simulink model "MCVT_v6_shell"  (R2021b)
settings: Solver=FixedStepAuto  StartTime=0.0  StopTime=1000000  FixedStep=1/fz  RelTol=1e-3
undefined symbols (not defined in the file or in its folder): fz_3
libraries: lib_subframe x71, slrealtimeutilitieslib x30, lib_header x15, slrealtimeiplib x15
(part 1 of 2)
settings Model: Creator=krishnan  LastModifiedBy=jiw19031
settings SolverCC: AlgebraicLoopSolver=TrustRegion
settings DebuggingCC: SFMachineParentedDataDiag=warning

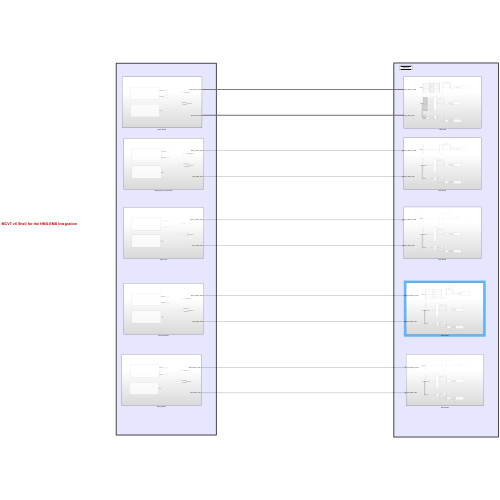
[thumbnail: Simulink's stored preview of the top-level diagram]
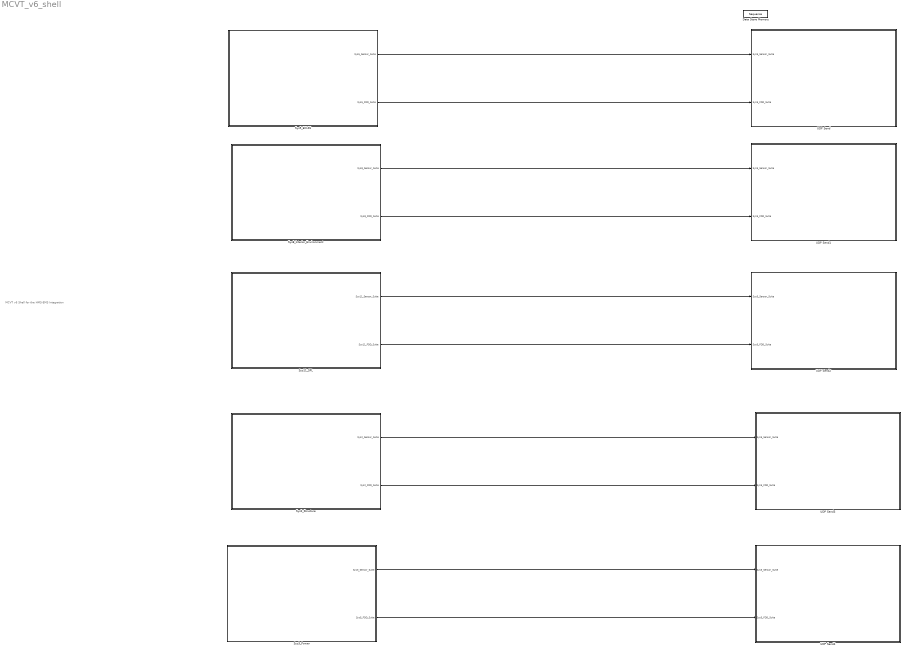
== system MCVT_v6_shell ==
  note: MCVT v6 Shell for the HMS-EMS Integration
  Data Store Memory : DataStoreMemory  DataStoreName=Sequence  ReadBeforeWriteMsg=warning  WriteAfterWriteMsg=warning  WriteAfterReadMsg=warning  ShowAdditionalParam=off  OutDataTypeStr=uint16
  Sys11_SPL : Subsystem
  Sys2_Structure : Subsystem
  Sys3_Power : Subsystem
  Sys5_ECLSS : Subsystem
  Sys8_Interior_Environment : Subsystem
  UDP Send : Subsystem
  UDP Send1 : Subsystem
  UDP Send2 : Subsystem
  UDP Send3 : Subsystem
  UDP Send4 : Subsystem
  wires:
  Sys5_ECLSS/1(Sys5_Sensor_Suite) -> UDP Send/1(Sys5_Sensor_Suite)
  Sys5_ECLSS/2(Sys5_FDD_Suite) -> UDP Send/2(Sys5_FDD_Suite)
  Sys8_Interior_Environment/1(Sys8_Sensor_Suite) -> UDP Send1/1(Sys5_Sensor_Suite)
  Sys8_Interior_Environment/2(Sys8_FDD_Suite) -> UDP Send1/2(Sys5_FDD_Suite)
  Sys11_SPL/1(Sys11_Sensor_Suite) -> UDP Send2/1(Sys5_Sensor_Suite)
  Sys11_SPL/2(Sys11_FDD_Suite) -> UDP Send2/2(Sys5_FDD_Suite)
  Sys2_Structure/1(Sys2_Sensor_Suite) -> UDP Send3/1(Sys5_Sensor_Suite)
  Sys2_Structure/2(Sys2_FDD_Suite) -> UDP Send3/2(Sys5_FDD_Suite)
  Sys3_Power/1(Sys3_Sensor_Suite) -> UDP Send4/1(Sys5_Sensor_Suite)
  Sys3_Power/2(Sys5_FDD_Suite) -> UDP Send4/2(Sys5_FDD_Suite)

== system MCVT_v6_shell/Sys11_SPL ==
  Bus Creator : BusCreator  Inputs=2
  Sys11_FDDs : Subsystem
  Sys11_Sensors : Subsystem
  Sys11_Sensor_Suite : Outport
  Sys11_FDD_Suite : Outport  Port=2
  wires:
  Sys11_Sensors/1(Sys8_Sensor_Measurements) -> [Sys11_Sensor_Suite]
  [Sys11_Sensor_Suite] -> Sys11_Sensor_Suite/1  "Sys11_Sensor_Suite"
  Sys11_Sensors/2(Sys8_Sensor_FDD_Measurements) -> [Sys11_Sensor_FDD]
  Sys11_FDDs/1(Sys11_Component_FDD_Suite) -> [Sys11_Component_FDD]
  [Sys11_Sensor_FDD] -> Bus Creator/1  "Sys11_Sensor_FDD"
  [Sys11_Component_FDD] -> Bus Creator/2  "Sys8_Component_FDD"
  Bus Creator/1 -> Sys11_FDD_Suite/1

== system MCVT_v6_shell/Sys2_Structure ==
  Bus Creator : BusCreator  Inputs=2
  Sys2_FDDs : Subsystem
  Sys2_Sensors : Subsystem
  Sys2_Sensor_Suite : Outport
  Sys2_FDD_Suite : Outport  Port=2
  wires:
  Sys2_Sensors/1(Sys2_Sensor_Measurements) -> [Sys2_Sensor_Suite]
  [Sys2_Sensor_Suite] -> Sys2_Sensor_Suite/1  "Sys2_Sensor_Suite"
  Sys2_Sensors/2(Sys2_Sensor_FDD_Measurements) -> [Sys2_Sensor_FDD]
  Sys2_FDDs/1(Sys2_Component_FDDs) -> [Sys2_Component_FDD]
  [Sys2_Sensor_FDD] -> Bus Creator/1  "Sys2_Sensor_FDD"
  [Sys2_Component_FDD] -> Bus Creator/2  "Sys2_Component_FDD"
  Bus Creator/1 -> Sys2_FDD_Suite/1  "Sys2_FDD_Suite"

== system MCVT_v6_shell/Sys3_Power ==
  Bus Creator : BusCreator  Inputs=2
  Sys3_FDDs : Subsystem
  Sys3_Sensors : Subsystem
  Sys3_Sensor_Suite : Outport
  Sys5_FDD_Suite : Outport  Port=2
  wires:
  Sys3_Sensors/1(Sys3_Sensor_Measurements) -> [Sys3_Sensor_Suite]
  [Sys3_Sensor_Suite] -> Sys3_Sensor_Suite/1  "Sys3_Sensor_Suite"
  Sys3_Sensors/2(Sys3_Sensor_FDD_Measurements) -> [Sys3_Sensor_FDD]
  Sys3_FDDs/1(Sys3_Component_FDDs) -> [Sys3_Component_FDD]
  [Sys3_Sensor_FDD] -> Bus Creator/1  "Sys3_Sensor_FDD"
  [Sys3_Component_FDD] -> Bus Creator/2  "Sys3_Component_FDD"
  Bus Creator/1 -> Sys5_FDD_Suite/1  "Sys3_FDD_Suite"

== system MCVT_v6_shell/Sys5_ECLSS ==
  Bus Creator : BusCreator  Inputs=2
  Sys5_FDDs : Subsystem
  Sys5_Sensors : Subsystem
  Sys5_Sensor_Suite : Outport
  Sys5_FDD_Suite : Outport  Port=2
  wires:
  Sys5_Sensors/1(Sys5_Sensor_Measurements) -> [Sys5_Sensor_Suite]
  [Sys5_Sensor_Suite] -> Sys5_Sensor_Suite/1  "Sys5_Sensor_Suite"
  Sys5_Sensors/2(Sys5_Sensor_FDD_Measurements) -> [Sys5_Sensor_FDD]
  Sys5_FDDs/1(Sys5_Component_FDDs) -> [Sys5_Component_FDD]
  [Sys5_Sensor_FDD] -> Bus Creator/1  "Sys5_Sensor_FDD"
  [Sys5_Component_FDD] -> Bus Creator/2  "Sys5_Component_FDD"
  Bus Creator/1 -> Sys5_FDD_Suite/1  "Sys5_FDD_Suite"

== system MCVT_v6_shell/Sys8_Interior_Environment ==
  Bus Creator : BusCreator  Inputs=2
  Sys8_FDDs : Subsystem
  Sys8_Sensors : Subsystem
  Sys8_Sensor_Suite : Outport
  Sys8_FDD_Suite : Outport  Port=2
  wires:
  Sys8_Sensors/1(Sys8_Sensor_Measurements) -> [Sys8_Sensor_Suite]
  [Sys8_Sensor_Suite] -> Sys8_Sensor_Suite/1  "Sys8_Sensor_Suite"
  Sys8_Sensors/2(Sys8_Sensor_FDD_Measurements) -> [Sys8_Sensor_FDD]
  Sys8_FDDs/1(Sys8_Component_FDD_Suite) -> [Sys8_Component_FDD]
  [Sys8_Sensor_FDD] -> Bus Creator/1  "Sys8_Sensor_FDD"
  [Sys8_Component_FDD] -> Bus Creator/2  "Sys8_Component_FDD"
  Bus Creator/1 -> Sys8_FDD_Suite/1  "Sys8_FDD_Suite"

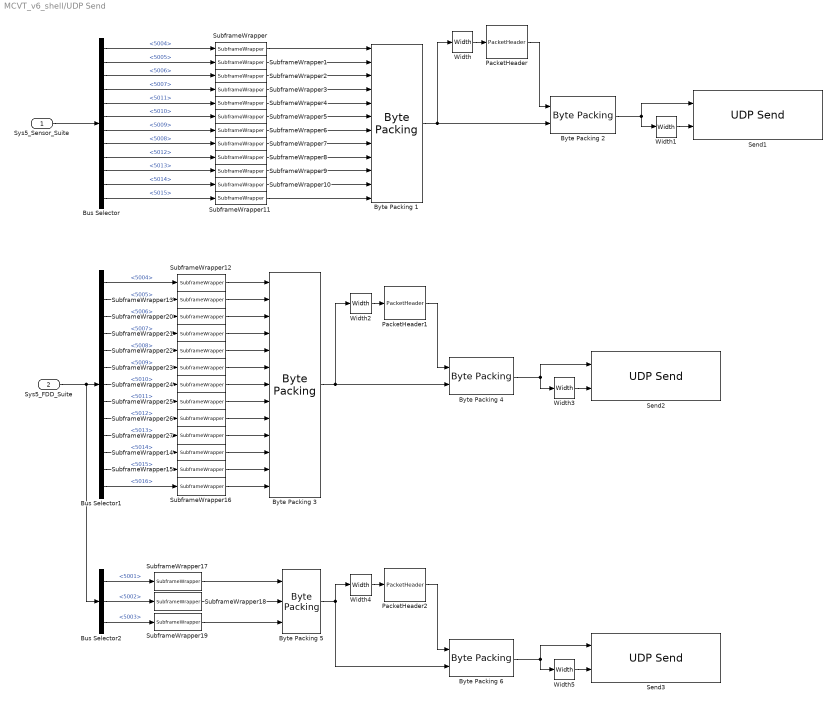
== system MCVT_v6_shell/UDP Send ==
  Sys5_Sensor_Suite : Inport
  Sys5_FDD_Suite : Inport  Port=2
  Bus Selector : BusSelector  OutputSignals=5004,5005,5006,5007,5011,5010,5009,5008,5012,5013,5014,5015
  Bus Selector1 : BusSelector  OutputSignals=Sys5_Sensor_FDD.5004,Sys5_Sensor_FDD.5005,Sys5_Sensor_FDD.5006,Sys5_Sensor_FDD.5007,Sys5_Sensor_FDD.5008,Sys5_Sensor_FDD.5009,Sys5_Sensor_FDD.5010,Sys5_Sensor_FDD.5011,Sys5_Sensor_FDD.5012,Sys5_Sensor_FDD.5013,Sys5_Sensor_FDD.5014,Sys5_Sensor_FDD.5015,Sys5_Sensor_FDD.5016
  Bus Selector2 : BusSelector  OutputSignals=Sys5_Component_FDD.5001,Sys5_Component_FDD.5002,Sys5_Component_FDD.5003
  Byte Packing {1..6} (6 alike) : slrealtimeutilitieslib/Byte Packing
  PacketHeader : lib_header/PacketHeader  src=4  dst=1  pkt_type=1  pkt_priority=1  service=0  flag=0  option1=0  option2=0  subframe_num=12
  PacketHeader1 : lib_header/PacketHeader  src=4  dst=1  pkt_type=1  pkt_priority=1  service=0  flag=0  option1=0  option2=0  subframe_num=13
  PacketHeader2 : lib_header/PacketHeader  src=4  dst=1  pkt_type=1  pkt_priority=1  service=0  flag=0  option1=0  option2=0  subframe_num=3
  Send1 : slrealtimeiplib/UDP Send  useHostTargetConn=on  toAddress=192.168.50.190  toPort=10004  sampleTime=1  localPort=-1
      settings: SourceProductBaseCode=XP
  Send2 : slrealtimeiplib/UDP Send  useHostTargetConn=on  toAddress=192.168.50.190  toPort=10004  sampleTime=1  localPort=-1
      settings: SourceProductBaseCode=XP
  Send3 : slrealtimeiplib/UDP Send  useHostTargetConn=on  toAddress=192.168.50.190  toPort=10004  sampleTime=1  localPort=-1
      settings: SourceProductBaseCode=XP
  SubframeWrapper : lib_subframe/SubframeWrapper  data_id=504
  SubframeWrapper1 : lib_subframe/SubframeWrapper  data_id=505
  SubframeWrapper10 : lib_subframe/SubframeWrapper  data_id=514
  SubframeWrapper11 : lib_subframe/SubframeWrapper  data_id=515
  SubframeWrapper12 : lib_subframe/SubframeWrapper  data_id=5004
  SubframeWrapper13 : lib_subframe/SubframeWrapper  data_id=5005
  SubframeWrapper14 : lib_subframe/SubframeWrapper  data_id=5014
  SubframeWrapper15 : lib_subframe/SubframeWrapper  data_id=5015
  SubframeWrapper16 : lib_subframe/SubframeWrapper  data_id=5016
  SubframeWrapper17 : lib_subframe/SubframeWrapper  data_id=5001
  SubframeWrapper18 : lib_subframe/SubframeWrapper  data_id=5002
  SubframeWrapper19 : lib_subframe/SubframeWrapper  data_id=5003
  SubframeWrapper2 : lib_subframe/SubframeWrapper  data_id=506
  SubframeWrapper20 : lib_subframe/SubframeWrapper  data_id=5006
  SubframeWrapper21 : lib_subframe/SubframeWrapper  data_id=5007
  SubframeWrapper22 : lib_subframe/SubframeWrapper  data_id=5008
  SubframeWrapper23 : lib_subframe/SubframeWrapper  data_id=5009
  SubframeWrapper24 : lib_subframe/SubframeWrapper  data_id=5010
  SubframeWrapper25 : lib_subframe/SubframeWrapper  data_id=5011
  SubframeWrapper26 : lib_subframe/SubframeWrapper  data_id=5012
  SubframeWrapper27 : lib_subframe/SubframeWrapper  data_id=5013
  SubframeWrapper3 : lib_subframe/SubframeWrapper  data_id=507
  SubframeWrapper4 : lib_subframe/SubframeWrapper  data_id=511
  SubframeWrapper5 : lib_subframe/SubframeWrapper  data_id=510
  SubframeWrapper6 : lib_subframe/SubframeWrapper  data_id=509
  SubframeWrapper7 : lib_subframe/SubframeWrapper  data_id=508
  SubframeWrapper8 : lib_subframe/SubframeWrapper  data_id=512
  SubframeWrapper9 : lib_subframe/SubframeWrapper  data_id=513
  Width{,1..5} (6 alike) : Width
  wires:
  Byte Packing 1/1 -> Byte Packing 2/2, Width/1
  Sys5_Sensor_Suite/1 -> Bus Selector/1
  Width/1 -> PacketHeader/1
  PacketHeader/1 -> Byte Packing 2/1
  Byte Packing 2/1 -> Width1/1, Send1/1
  Width1/1 -> Send1/2
  Bus Selector/1 -> SubframeWrapper/1  "<5004>"
  Bus Selector/2 -> SubframeWrapper1/1  "<5005>"
  Bus Selector/3 -> SubframeWrapper2/1  "<5006>"
  Bus Selector/4 -> SubframeWrapper3/1  "<5007>"
  Bus Selector/5 -> SubframeWrapper4/1  "<5011>"
  Bus Selector/6 -> SubframeWrapper5/1  "<5010>"
  Bus Selector/7 -> SubframeWrapper6/1  "<5009>"
  Bus Selector/8 -> SubframeWrapper7/1  "<5008>"
  Bus Selector/9 -> SubframeWrapper8/1  "<5012>"
  Bus Selector/10 -> SubframeWrapper9/1  "<5013>"
  Bus Selector/11 -> SubframeWrapper10/1  "<5014>"
  Bus Selector/12 -> SubframeWrapper11/1  "<5015>"
  SubframeWrapper/1 -> Byte Packing 1/1
  SubframeWrapper1/1 -> Byte Packing 1/2
  SubframeWrapper2/1 -> Byte Packing 1/3
  SubframeWrapper3/1 -> Byte Packing 1/4
  SubframeWrapper4/1 -> Byte Packing 1/5
  SubframeWrapper5/1 -> Byte Packing 1/6
  SubframeWrapper6/1 -> Byte Packing 1/7
  SubframeWrapper7/1 -> Byte Packing 1/8
  SubframeWrapper8/1 -> Byte Packing 1/9
  SubframeWrapper9/1 -> Byte Packing 1/10
  SubframeWrapper10/1 -> Byte Packing 1/11
  SubframeWrapper11/1 -> Byte Packing 1/12
  Bus Selector2/2 -> SubframeWrapper18/1  "<5002>"
  Byte Packing 6/1 -> Width5/1, Send3/1
  SubframeWrapper18/1 -> Byte Packing 5/2
  Bus Selector1/8 -> SubframeWrapper25/1  "<5011>"
  PacketHeader2/1 -> Byte Packing 6/1
  SubframeWrapper17/1 -> Byte Packing 5/1
  Bus Selector1/11 -> SubframeWrapper14/1  "<5014>"
  SubframeWrapper14/1 -> Byte Packing 3/11
  SubframeWrapper27/1 -> Byte Packing 3/10
  Bus Selector1/4 -> SubframeWrapper21/1  "<5007>"
  SubframeWrapper19/1 -> Byte Packing 5/3
  SubframeWrapper15/1 -> Byte Packing 3/12
  SubframeWrapper16/1 -> Byte Packing 3/13
  Bus Selector2/3 -> SubframeWrapper19/1  "<5003>"
  Byte Packing 5/1 -> Byte Packing 6/2, Width4/1
  SubframeWrapper25/1 -> Byte Packing 3/8
  Width4/1 -> PacketHeader2/1
  SubframeWrapper26/1 -> Byte Packing 3/9
  Bus Selector2/1 -> SubframeWrapper17/1  "<5001>"
  Bus Selector1/7 -> SubframeWrapper24/1  "<5010>"
  SubframeWrapper12/1 -> Byte Packing 3/1
  Bus Selector1/10 -> SubframeWrapper27/1  "<5013>"
  Bus Selector1/9 -> SubframeWrapper26/1  "<5012>"
  Bus Selector1/12 -> SubframeWrapper15/1  "<5015>"
  Byte Packing 3/1 -> Byte Packing 4/2, Width2/1
  Bus Selector1/13 -> SubframeWrapper16/1  "<5016>"
  SubframeWrapper24/1 -> Byte Packing 3/7
  SubframeWrapper23/1 -> Byte Packing 3/6
  SubframeWrapper21/1 -> Byte Packing 3/4
  SubframeWrapper20/1 -> Byte Packing 3/3
  Bus Selector1/2 -> SubframeWrapper13/1  "<5005>"
  SubframeWrapper22/1 -> Byte Packing 3/5
  SubframeWrapper13/1 -> Byte Packing 3/2
  Width2/1 -> PacketHeader1/1
  Width3/1 -> Send2/2
  Bus Selector1/1 -> SubframeWrapper12/1  "<5004>"
  Bus Selector1/3 -> SubframeWrapper20/1  "<5006>"
  Bus Selector1/5 -> SubframeWrapper22/1  "<5008>"
  Sys5_FDD_Suite/1 -> Bus Selector2/1, Bus Selector1/1
  Byte Packing 4/1 -> Width3/1, Send2/1
  Width5/1 -> Send3/2
  PacketHeader1/1 -> Byte Packing 4/1
  Bus Selector1/6 -> SubframeWrapper23/1  "<5009>"

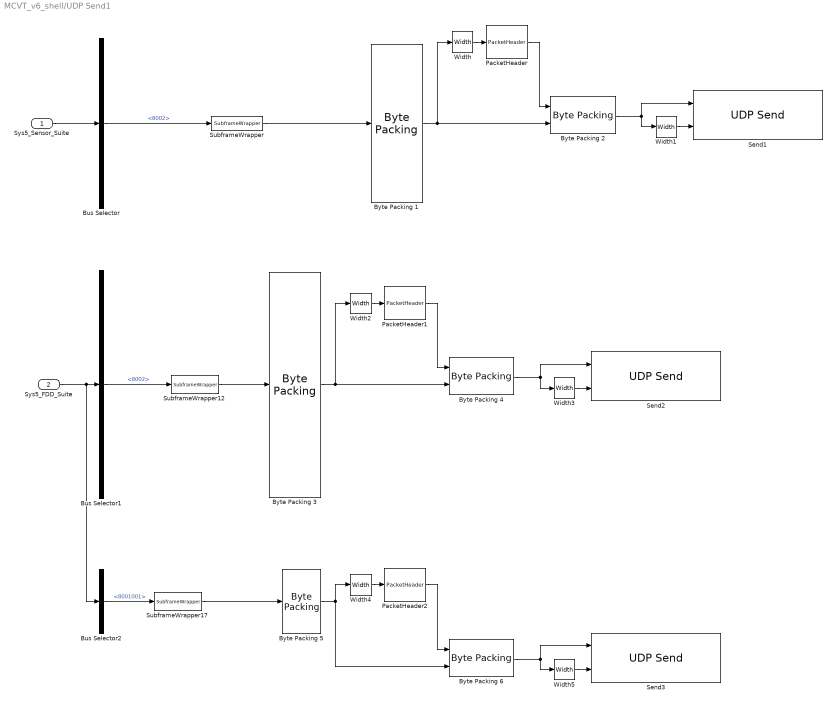
== system MCVT_v6_shell/UDP Send1 ==
  Sys5_Sensor_Suite : Inport
  Sys5_FDD_Suite : Inport  Port=2
  Bus Selector : BusSelector  OutputSignals=8002
  Bus Selector1 : BusSelector  OutputSignals=Sys8_Sensor_FDD.8002
  Bus Selector2 : BusSelector  OutputSignals=Sys8_Component_FDD.8001001
  Byte Packing {1..6} (6 alike) : slrealtimeutilitieslib/Byte Packing
  PacketHeader : lib_header/PacketHeader  src=6  dst=1  pkt_type=1  pkt_priority=1  service=0  flag=0  option1=0  option2=0  subframe_num=1
  PacketHeader1 : lib_header/PacketHeader  src=6  dst=1  pkt_type=1  pkt_priority=1  service=0  flag=0  option1=0  option2=0  subframe_num=1
  PacketHeader2 : lib_header/PacketHeader  src=6  dst=1  pkt_type=1  pkt_priority=1  service=0  flag=0  option1=0  option2=0  subframe_num=1
  Send1 : slrealtimeiplib/UDP Send  useHostTargetConn=on  toAddress=192.168.50.190  toPort=10006  sampleTime=1  localPort=-1
      settings: SourceProductBaseCode=XP
  Send2 : slrealtimeiplib/UDP Send  useHostTargetConn=on  toAddress=192.168.50.190  toPort=10006  sampleTime=1  localPort=-1
      settings: SourceProductBaseCode=XP
  Send3 : slrealtimeiplib/UDP Send  useHostTargetConn=on  toAddress=192.168.50.190  toPort=10006  sampleTime=1  localPort=-1
      settings: SourceProductBaseCode=XP
  SubframeWrapper : lib_subframe/SubframeWrapper  data_id=802
  SubframeWrapper12 : lib_subframe/SubframeWrapper  data_id=8002
  SubframeWrapper17 : lib_subframe/SubframeWrapper  data_id=8001
  Width{,1..5} (6 alike) : Width
  wires:
  Byte Packing 1/1 -> Byte Packing 2/2, Width/1
  Sys5_Sensor_Suite/1 -> Bus Selector/1
  Width/1 -> PacketHeader/1
  PacketHeader/1 -> Byte Packing 2/1
  Byte Packing 2/1 -> Width1/1, Send1/1
  Width1/1 -> Send1/2
  Bus Selector/1 -> SubframeWrapper/1  "<8002>"
  SubframeWrapper/1 -> Byte Packing 1/1
  Byte Packing 6/1 -> Width5/1, Send3/1
  PacketHeader2/1 -> Byte Packing 6/1
  SubframeWrapper17/1 -> Byte Packing 5/1
  Byte Packing 5/1 -> Byte Packing 6/2, Width4/1
  Width4/1 -> PacketHeader2/1
  Bus Selector2/1 -> SubframeWrapper17/1  "<8001001>"
  SubframeWrapper12/1 -> Byte Packing 3/1
  Byte Packing 3/1 -> Byte Packing 4/2, Width2/1
  Width2/1 -> PacketHeader1/1
  Width3/1 -> Send2/2
  Bus Selector1/1 -> SubframeWrapper12/1  "<8002>"
  Sys5_FDD_Suite/1 -> Bus Selector2/1, Bus Selector1/1
  Byte Packing 4/1 -> Width3/1, Send2/1
  Width5/1 -> Send3/2
  PacketHeader1/1 -> Byte Packing 4/1

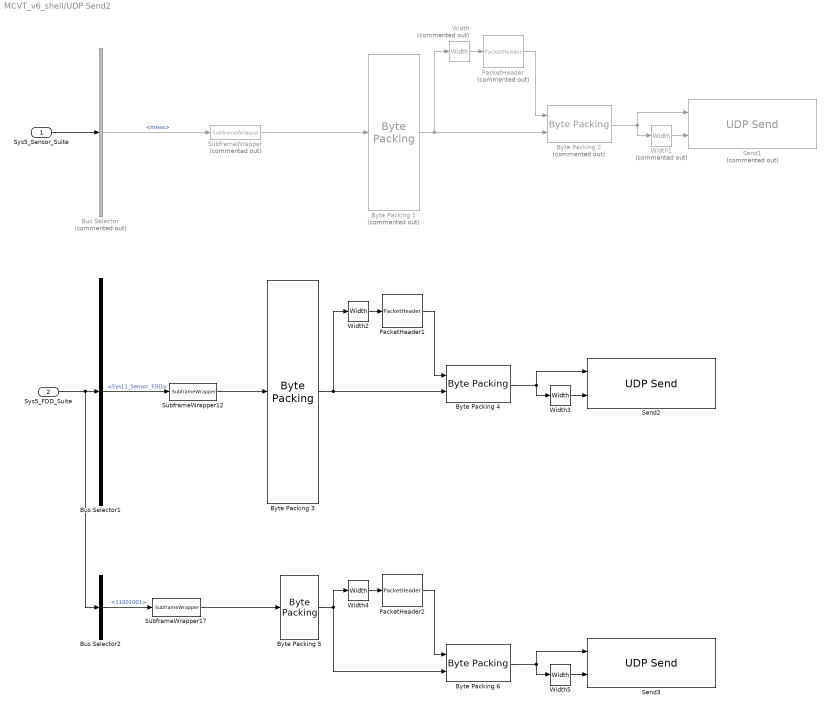
== system MCVT_v6_shell/UDP Send2 ==
  Sys5_Sensor_Suite : Inport
  Sys5_FDD_Suite : Inport  Port=2
  Bus Selector : BusSelector  Commented=on  OutputSignals=meas
  Bus Selector1 : BusSelector  OutputSignals=Sys11_Sensor_FDD
  Bus Selector2 : BusSelector  OutputSignals=Sys8_Component_FDD.11001001
  Byte Packing 1 : slrealtimeutilitieslib/Byte Packing  Commented=on  MaskPackedDataType=uint8  MaskUnpackedDataTypes={'uint8'}  MaskAlignment=1
  Byte Packing 2 : slrealtimeutilitieslib/Byte Packing  Commented=on  MaskPackedDataType=uint8  MaskUnpackedDataTypes={'uint8','uint8'}  MaskAlignment=1
  Byte Packing {3..6} (4 alike) : slrealtimeutilitieslib/Byte Packing
  PacketHeader : lib_header/PacketHeader  Commented=on  src=6  dst=1  pkt_type=1  pkt_priority=1  service=0  flag=0  option1=0  option2=0  subframe_num=1
  PacketHeader1 : lib_header/PacketHeader  src=8  dst=1  pkt_type=1  pkt_priority=1  service=0  flag=0  option1=0  option2=0  subframe_num=1
  PacketHeader2 : lib_header/PacketHeader  src=8  dst=1  pkt_type=1  pkt_priority=1  service=0  flag=0  option1=0  option2=0  subframe_num=1
  Send1 : slrealtimeiplib/UDP Send  Commented=on  useHostTargetConn=on  toAddress=192.168.50.190  toPort=10006  sampleTime=1  localPort=-1
      settings: SourceProductBaseCode=XP
  Send2 : slrealtimeiplib/UDP Send  useHostTargetConn=on  toAddress=192.168.50.190  toPort=10008  sampleTime=1  localPort=-1
      settings: SourceProductBaseCode=XP
  Send3 : slrealtimeiplib/UDP Send  useHostTargetConn=on  toAddress=192.168.50.190  toPort=10008  sampleTime=1  localPort=-1
      settings: SourceProductBaseCode=XP
  SubframeWrapper : lib_subframe/SubframeWrapper  Commented=on  data_id=1+128
  SubframeWrapper12 : lib_subframe/SubframeWrapper  data_id=5004
  SubframeWrapper17 : lib_subframe/SubframeWrapper  data_id=5001
  Width : Width  Commented=on
  Width1 : Width  Commented=on
  Width{2..5} (4 alike) : Width
  wires:
  Byte Packing 1/1 -> Byte Packing 2/2, Width/1
  Sys5_Sensor_Suite/1 -> Bus Selector/1
  Width/1 -> PacketHeader/1
  PacketHeader/1 -> Byte Packing 2/1
  Byte Packing 2/1 -> Width1/1, Send1/1
  Width1/1 -> Send1/2
  Bus Selector/1 -> SubframeWrapper/1  "<meas>"
  SubframeWrapper/1 -> Byte Packing 1/1
  Byte Packing 6/1 -> Width5/1, Send3/1
  PacketHeader2/1 -> Byte Packing 6/1
  SubframeWrapper17/1 -> Byte Packing 5/1
  Byte Packing 5/1 -> Byte Packing 6/2, Width4/1
  Width4/1 -> PacketHeader2/1
  Bus Selector2/1 -> SubframeWrapper17/1  "<11001001>"
  SubframeWrapper12/1 -> Byte Packing 3/1
  Byte Packing 3/1 -> Byte Packing 4/2, Width2/1
  Width2/1 -> PacketHeader1/1
  Width3/1 -> Send2/2
  Bus Selector1/1 -> SubframeWrapper12/1  "<Sys11_Sensor_FDD>"
  Sys5_FDD_Suite/1 -> Bus Selector2/1, Bus Selector1/1
  Byte Packing 4/1 -> Width3/1, Send2/1
  Width5/1 -> Send3/2
  PacketHeader1/1 -> Byte Packing 4/1

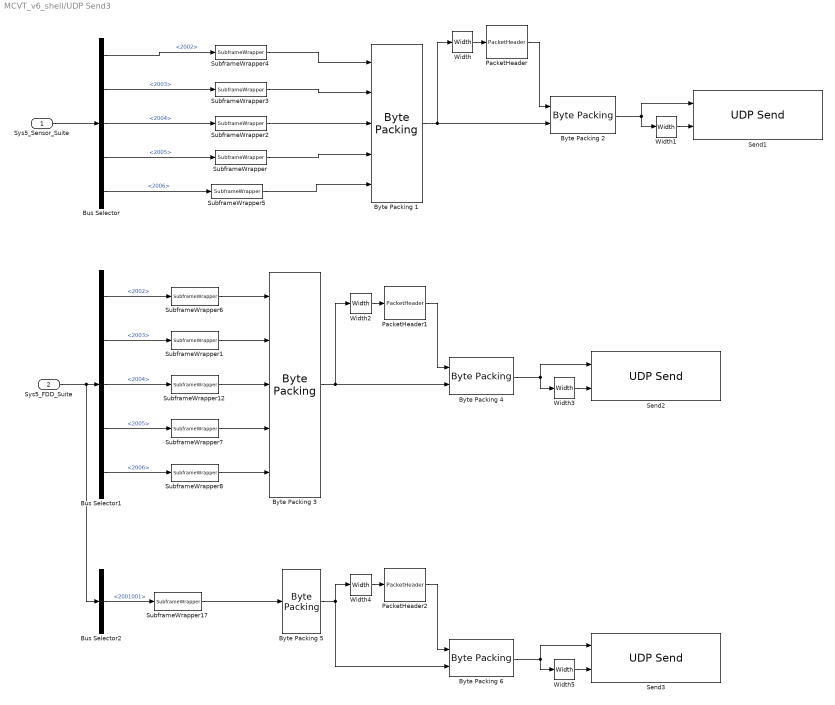
== system MCVT_v6_shell/UDP Send3 ==
  Sys5_Sensor_Suite : Inport
  Sys5_FDD_Suite : Inport  Port=2
  Bus Selector : BusSelector  OutputSignals=2002,2003,2004,2005,2006
  Bus Selector1 : BusSelector  OutputSignals=Sys2_Sensor_FDD.2002,Sys2_Sensor_FDD.2003,Sys2_Sensor_FDD.2004,Sys2_Sensor_FDD.2005,Sys2_Sensor_FDD.2006
  Bus Selector2 : BusSelector  OutputSignals=Sys2_Component_FDD.2001001
  Byte Packing {1..6} (6 alike) : slrealtimeutilitieslib/Byte Packing
  PacketHeader : lib_header/PacketHeader  src=6  dst=2  pkt_type=1  pkt_priority=1  service=0  flag=0  option1=0  option2=0  subframe_num=5
  PacketHeader1 : lib_header/PacketHeader  src=8  dst=2  pkt_type=1  pkt_priority=1  service=0  flag=0  option1=0  option2=0  subframe_num=5
  PacketHeader2 : lib_header/PacketHeader  src=8  dst=2  pkt_type=1  pkt_priority=1  service=0  flag=0  option1=0  option2=0  subframe_num=1
  Send1 : slrealtimeiplib/UDP Send  useHostTargetConn=on  toAddress=192.168.50.190  toPort=10002  sampleTime=1  localPort=-1
      settings: SourceProductBaseCode=XP
  Send2 : slrealtimeiplib/UDP Send  useHostTargetConn=on  toAddress=192.168.50.190  toPort=10002  sampleTime=1  localPort=-1
      settings: SourceProductBaseCode=XP
  Send3 : slrealtimeiplib/UDP Send  useHostTargetConn=on  toAddress=192.168.50.190  toPort=10002  sampleTime=1  localPort=-1
      settings: SourceProductBaseCode=XP
  SubframeWrapper : lib_subframe/SubframeWrapper  data_id=205
  SubframeWrapper1 : lib_subframe/SubframeWrapper  data_id=2003
  SubframeWrapper12 : lib_subframe/SubframeWrapper  data_id=2004
  SubframeWrapper17 : lib_subframe/SubframeWrapper  data_id=2001
  SubframeWrapper2 : lib_subframe/SubframeWrapper  data_id=204
  SubframeWrapper3 : lib_subframe/SubframeWrapper  data_id=203
  SubframeWrapper4 : lib_subframe/SubframeWrapper  data_id=202
  SubframeWrapper5 : lib_subframe/SubframeWrapper  data_id=206
  SubframeWrapper6 : lib_subframe/SubframeWrapper  data_id=2002
  SubframeWrapper7 : lib_subframe/SubframeWrapper  data_id=2005
  SubframeWrapper8 : lib_subframe/SubframeWrapper  data_id=2006
  Width{,1..5} (6 alike) : Width
  wires:
  Byte Packing 1/1 -> Byte Packing 2/2, Width/1
  Sys5_Sensor_Suite/1 -> Bus Selector/1
  Width/1 -> PacketHeader/1
  PacketHeader/1 -> Byte Packing 2/1
  Byte Packing 2/1 -> Width1/1, Send1/1
  Width1/1 -> Send1/2
  Byte Packing 6/1 -> Width5/1, Send3/1
  PacketHeader2/1 -> Byte Packing 6/1
  SubframeWrapper17/1 -> Byte Packing 5/1
  Byte Packing 5/1 -> Byte Packing 6/2, Width4/1
  Width4/1 -> PacketHeader2/1
  Bus Selector2/1 -> SubframeWrapper17/1  "<2001001>"
  Byte Packing 3/1 -> Byte Packing 4/2, Width2/1
  Width2/1 -> PacketHeader1/1
  Width3/1 -> Send2/2
  Sys5_FDD_Suite/1 -> Bus Selector2/1, Bus Selector1/1
  Byte Packing 4/1 -> Width3/1, Send2/1
  Width5/1 -> Send3/2
  PacketHeader1/1 -> Byte Packing 4/1
  Bus Selector/1 -> SubframeWrapper4/1  "<2002>"
  Bus Selector/2 -> SubframeWrapper3/1  "<2003>"
  Bus Selector/3 -> SubframeWrapper2/1  "<2004>"
  Bus Selector/4 -> SubframeWrapper/1  "<2005>"
  Bus Selector/5 -> SubframeWrapper5/1  "<2006>"
  SubframeWrapper4/1 -> Byte Packing 1/1
  SubframeWrapper3/1 -> Byte Packing 1/2
  SubframeWrapper2/1 -> Byte Packing 1/3
  SubframeWrapper/1 -> Byte Packing 1/4
  SubframeWrapper5/1 -> Byte Packing 1/5
  Bus Selector1/1 -> SubframeWrapper6/1  "<2002>"
  Bus Selector1/2 -> SubframeWrapper1/1  "<2003>"
  Bus Selector1/3 -> SubframeWrapper12/1  "<2004>"
  Bus Selector1/4 -> SubframeWrapper7/1  "<2005>"
  Bus Selector1/5 -> SubframeWrapper8/1  "<2006>"
  SubframeWrapper6/1 -> Byte Packing 3/1
  SubframeWrapper1/1 -> Byte Packing 3/2
  SubframeWrapper12/1 -> Byte Packing 3/3
  SubframeWrapper7/1 -> Byte Packing 3/4
  SubframeWrapper8/1 -> Byte Packing 3/5

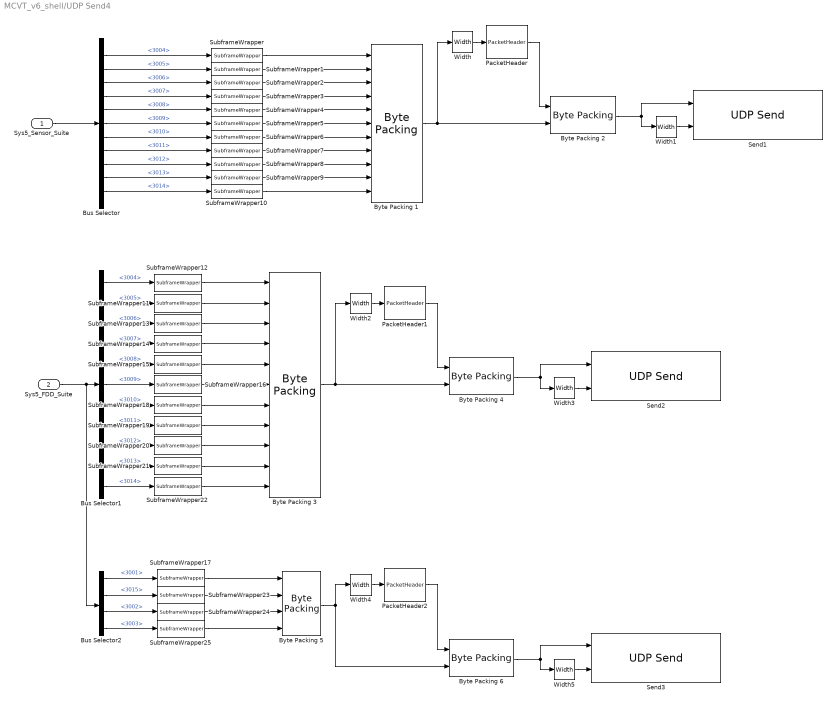
== system MCVT_v6_shell/UDP Send4 ==
  Sys5_Sensor_Suite : Inport
  Sys5_FDD_Suite : Inport  Port=2
  Bus Selector : BusSelector  OutputSignals=3004,3005,3006,3007,3008,3009,3010,3011,3012,3013,3014
  Bus Selector1 : BusSelector  OutputSignals=Sys3_Sensor_FDD.3004,Sys3_Sensor_FDD.3005,Sys3_Sensor_FDD.3006,Sys3_Sensor_FDD.3007,Sys3_Sensor_FDD.3008,Sys3_Sensor_FDD.3009,Sys3_Sensor_FDD.3010,Sys3_Sensor_FDD.3011,Sys3_Sensor_FDD.3012,Sys3_Sensor_FDD.3013,Sys3_Sensor_FDD.3014
  Bus Selector2 : BusSelector  OutputSignals=Sys3_Component_FDD.3001,Sys3_Component_FDD.3015,Sys3_Component_FDD.3002,Sys3_Component_FDD.3003
  Byte Packing {1..6} (6 alike) : slrealtimeutilitieslib/Byte Packing
  PacketHeader : lib_header/PacketHeader  src=3  dst=1  pkt_type=1  pkt_priority=1  service=0  flag=0  option1=0  option2=0  subframe_num=11
  PacketHeader1 : lib_header/PacketHeader  src=3  dst=1  pkt_type=1  pkt_priority=1  service=0  flag=0  option1=0  option2=0  subframe_num=11
  PacketHeader2 : lib_header/PacketHeader  src=3  dst=1  pkt_type=1  pkt_priority=1  service=0  flag=0  option1=0  option2=0  subframe_num=4
  Send1 : slrealtimeiplib/UDP Send  useHostTargetConn=on  toAddress=192.168.50.190  toPort=10003  sampleTime=1  localPort=-1
      settings: SourceProductBaseCode=XP
  Send2 : slrealtimeiplib/UDP Send  useHostTargetConn=on  toAddress=192.168.50.190  toPort=10003  sampleTime=1  localPort=-1
      settings: SourceProductBaseCode=XP
  Send3 : slrealtimeiplib/UDP Send  useHostTargetConn=on  toAddress=192.168.50.190  toPort=10003  sampleTime=1  localPort=-1
      settings: SourceProductBaseCode=XP
  SubframeWrapper : lib_subframe/SubframeWrapper  data_id=304
  SubframeWrapper1 : lib_subframe/SubframeWrapper  data_id=305
  SubframeWrapper10 : lib_subframe/SubframeWrapper  data_id=314
  SubframeWrapper11 : lib_subframe/SubframeWrapper  data_id=3005
  SubframeWrapper12 : lib_subframe/SubframeWrapper  data_id=3004
  SubframeWrapper13 : lib_subframe/SubframeWrapper  data_id=3006
  SubframeWrapper14 : lib_subframe/SubframeWrapper  data_id=3007
  SubframeWrapper15 : lib_subframe/SubframeWrapper  data_id=3008
  SubframeWrapper16 : lib_subframe/SubframeWrapper  data_id=3009
  SubframeWrapper17 : lib_subframe/SubframeWrapper  data_id=3001
  SubframeWrapper18 : lib_subframe/SubframeWrapper  data_id=3010
  SubframeWrapper19 : lib_subframe/SubframeWrapper  data_id=3011
  SubframeWrapper2 : lib_subframe/SubframeWrapper  data_id=306
  SubframeWrapper20 : lib_subframe/SubframeWrapper  data_id=3012
  SubframeWrapper21 : lib_subframe/SubframeWrapper  data_id=3013
  SubframeWrapper22 : lib_subframe/SubframeWrapper  data_id=3014
  SubframeWrapper23 : lib_subframe/SubframeWrapper  data_id=3015
  SubframeWrapper24 : lib_subframe/SubframeWrapper  data_id=3002
  SubframeWrapper25 : lib_subframe/SubframeWrapper  data_id=3003
  SubframeWrapper3 : lib_subframe/SubframeWrapper  data_id=307
  SubframeWrapper4 : lib_subframe/SubframeWrapper  data_id=308
  SubframeWrapper5 : lib_subframe/SubframeWrapper  data_id=309
  SubframeWrapper6 : lib_subframe/SubframeWrapper  data_id=310
  SubframeWrapper7 : lib_subframe/SubframeWrapper  data_id=311
  SubframeWrapper8 : lib_subframe/SubframeWrapper  data_id=312
  SubframeWrapper9 : lib_subframe/SubframeWrapper  data_id=313
  Width{,1..5} (6 alike) : Width
  wires:
  Byte Packing 1/1 -> Byte Packing 2/2, Width/1
  Sys5_Sensor_Suite/1 -> Bus Selector/1
  Width/1 -> PacketHeader/1
  PacketHeader/1 -> Byte Packing 2/1
  Byte Packing 2/1 -> Width1/1, Send1/1
  Width1/1 -> Send1/2
  Byte Packing 6/1 -> Width5/1, Send3/1
  PacketHeader2/1 -> Byte Packing 6/1
  Byte Packing 5/1 -> Width4/1, Byte Packing 6/2
  Width4/1 -> PacketHeader2/1
  Byte Packing 3/1 -> Byte Packing 4/2, Width2/1
  Width2/1 -> PacketHeader1/1
  Width3/1 -> Send2/2
  Sys5_FDD_Suite/1 -> Bus Selector2/1, Bus Selector1/1
  Byte Packing 4/1 -> Width3/1, Send2/1
  Width5/1 -> Send3/2
  PacketHeader1/1 -> Byte Packing 4/1
  Bus Selector/2 -> SubframeWrapper1/1  "<3005>"
  Bus Selector/1 -> SubframeWrapper/1  "<3004>"
  Bus Selector/3 -> SubframeWrapper2/1  "<3006>"
  Bus Selector/4 -> SubframeWrapper3/1  "<3007>"
  Bus Selector/5 -> SubframeWrapper4/1  "<3008>"
  Bus Selector/6 -> SubframeWrapper5/1  "<3009>"
  Bus Selector/7 -> SubframeWrapper6/1  "<3010>"
  Bus Selector/8 -> SubframeWrapper7/1  "<3011>"
  Bus Selector/9 -> SubframeWrapper8/1  "<3012>"
  Bus Selector/10 -> SubframeWrapper9/1  "<3013>"
  Bus Selector/11 -> SubframeWrapper10/1  "<3014>"
  SubframeWrapper/1 -> Byte Packing 1/1
  SubframeWrapper1/1 -> Byte Packing 1/2
  SubframeWrapper2/1 -> Byte Packing 1/3
  SubframeWrapper3/1 -> Byte Packing 1/4
  SubframeWrapper4/1 -> Byte Packing 1/5
  SubframeWrapper5/1 -> Byte Packing 1/6
  SubframeWrapper6/1 -> Byte Packing 1/7
  SubframeWrapper7/1 -> Byte Packing 1/8
  SubframeWrapper8/1 -> Byte Packing 1/9
  SubframeWrapper9/1 -> Byte Packing 1/10
  SubframeWrapper10/1 -> Byte Packing 1/11
  Bus Selector1/1 -> SubframeWrapper12/1  "<3004>"
  Bus Selector1/2 -> SubframeWrapper11/1  "<3005>"
  Bus Selector1/3 -> SubframeWrapper13/1  "<3006>"
  Bus Selector1/4 -> SubframeWrapper14/1  "<3007>"
  Bus Selector1/5 -> SubframeWrapper15/1  "<3008>"
  Bus Selector1/6 -> SubframeWrapper16/1  "<3009>"
  Bus Selector1/7 -> SubframeWrapper18/1  "<3010>"
  Bus Selector1/8 -> SubframeWrapper19/1  "<3011>"
  Bus Selector1/9 -> SubframeWrapper20/1  "<3012>"
  Bus Selector1/10 -> SubframeWrapper21/1  "<3013>"
  Bus Selector1/11 -> SubframeWrapper22/1  "<3014>"
  SubframeWrapper12/1 -> Byte Packing 3/1
  SubframeWrapper11/1 -> Byte Packing 3/2
  SubframeWrapper13/1 -> Byte Packing 3/3
  SubframeWrapper14/1 -> Byte Packing 3/4
  SubframeWrapper15/1 -> Byte Packing 3/5
  SubframeWrapper16/1 -> Byte Packing 3/6
  SubframeWrapper18/1 -> Byte Packing 3/7
  SubframeWrapper19/1 -> Byte Packing 3/8
  SubframeWrapper20/1 -> Byte Packing 3/9
  SubframeWrapper21/1 -> Byte Packing 3/10
  SubframeWrapper22/1 -> Byte Packing 3/11
  Bus Selector2/1 -> SubframeWrapper17/1  "<3001>"
  Bus Selector2/2 -> SubframeWrapper23/1  "<3015>"
  Bus Selector2/3 -> SubframeWrapper24/1  "<3002>"
  Bus Selector2/4 -> SubframeWrapper25/1  "<3003>"
  SubframeWrapper17/1 -> Byte Packing 5/1
  SubframeWrapper23/1 -> Byte Packing 5/2
  SubframeWrapper24/1 -> Byte Packing 5/3
  SubframeWrapper25/1 -> Byte Packing 5/4

== system MCVT_v6_shell/Sys11_SPL/Sys11_FDDs ==
  11001001 : MATLAB Function  TreatAsAtomicUnit=on
  Bus Creator : BusCreator  Inputs=1
  Sys11_Component_FDD_Suite : Outport
  wires:
  11001001/1(fddmeas) -> [FDDMEAS_11001001]  "11001001"
  [FDDMEAS_11001001] -> Bus Creator/1
  Bus Creator/1 -> Sys11_Component_FDD_Suite/1  "11001"

== system MCVT_v6_shell/Sys11_SPL/Sys11_Sensors ==
  Sys8_Sensor_Measurements : Outport
  Sys8_Sensor_FDD_Measurements : Outport  Port=2

== system MCVT_v6_shell/Sys2_Structure/Sys2_FDDs ==
  2001001 : MATLAB Function  TreatAsAtomicUnit=on
  Bus Creator : BusCreator  Inputs=1
  Sys2_Component_FDDs : Outport
  wires:
  2001001/1(fddmeas) -> [FDDMEAS_2001001]  "2001001"
  [FDDMEAS_2001001] -> Bus Creator/1
  Bus Creator/1 -> Sys2_Component_FDDs/1  "2001"

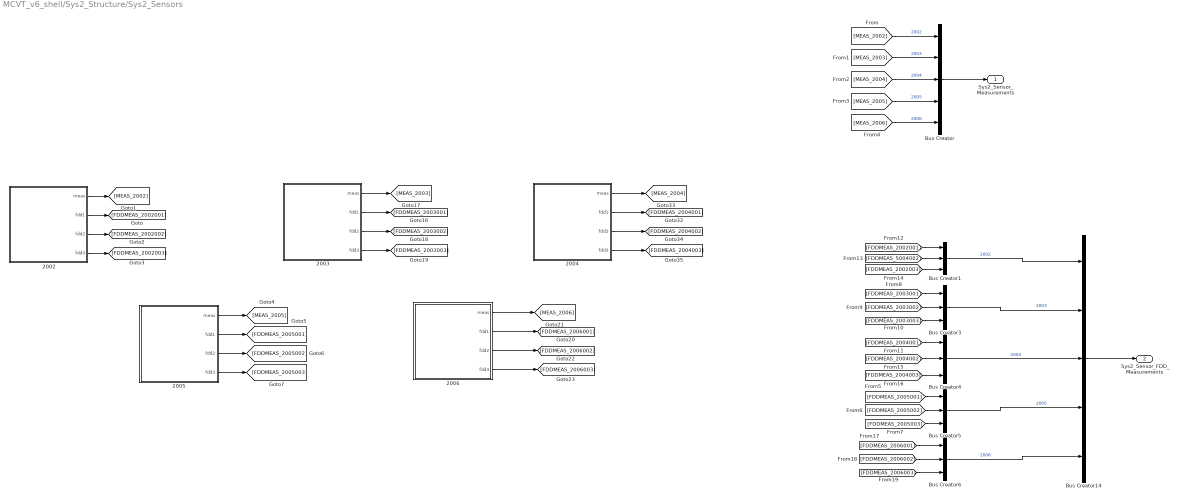
== system MCVT_v6_shell/Sys2_Structure/Sys2_Sensors ==
  2002 : MATLAB Function  TreatAsAtomicUnit=on
  2003 : MATLAB Function  TreatAsAtomicUnit=on
  2004 : MATLAB Function  TreatAsAtomicUnit=on
  2005 : MATLAB Function  TreatAsAtomicUnit=on
  2006 : MATLAB Function  TreatAsAtomicUnit=on
  Bus Creator : BusCreator  Inputs=5
  Bus Creator{1,3..6} (5 alike) : BusCreator  Inputs=3
  Bus Creator14 : BusCreator  Inputs=5
  Sys2_Sensor_Measurements : Outport
  Sys2_Sensor_FDD_Measurements : Outport  Port=2
  wires:
  Bus Creator/1 -> Sys2_Sensor_Measurements/1
  2002/1(meas) -> [MEAS_2002]
  2002/2(fdd1) -> [FDDMEAS_2002001]
  2002/3(fdd2) -> [FDDMEAS_2002002]
  2002/4(fdd3) -> [FDDMEAS_2002003]
  2005/1(meas) -> [MEAS_2005]
  2005/2(fdd1) -> [FDDMEAS_2005001]
  2005/3(fdd2) -> [FDDMEAS_2005002]
  2005/4(fdd3) -> [FDDMEAS_2005003]
  2003/1(meas) -> [MEAS_2003]
  2003/2(fdd1) -> [FDDMEAS_2003001]
  2003/3(fdd2) -> [FDDMEAS_2003002]
  2003/4(fdd3) -> [FDDMEAS_2003003]
  2006/1(meas) -> [MEAS_2006]
  2006/2(fdd1) -> [FDDMEAS_2006001]
  2006/3(fdd2) -> [FDDMEAS_2006002]
  2006/4(fdd3) -> [FDDMEAS_2006003]
  2004/1(meas) -> [MEAS_2004]
  2004/2(fdd1) -> [FDDMEAS_2004001]
  2004/3(fdd2) -> [FDDMEAS_2004002]
  2004/4(fdd3) -> [FDDMEAS_2004003]
  [MEAS_2002] -> Bus Creator/1  "2002"
  [FDDMEAS_2002001] -> Bus Creator1/1
  [FDDMEAS_5004002] -> Bus Creator1/2
  [FDDMEAS_2002003] -> Bus Creator1/3
  Bus Creator1/1 -> Bus Creator14/1  "2002"
  Bus Creator3/1 -> Bus Creator14/2  "2003"
  Bus Creator4/1 -> Bus Creator14/3  "2004"
  Bus Creator5/1 -> Bus Creator14/4  "2005"
  Bus Creator6/1 -> Bus Creator14/5  "2006"
  Bus Creator14/1 -> Sys2_Sensor_FDD_Measurements/1
  [MEAS_2003] -> Bus Creator/2  "2003"
  [MEAS_2004] -> Bus Creator/3  "2004"
  [MEAS_2005] -> Bus Creator/4  "2005"
  [MEAS_2006] -> Bus Creator/5  "2006"
  [FDDMEAS_2005001] -> Bus Creator5/1
  [FDDMEAS_2005002] -> Bus Creator5/2
  [FDDMEAS_2005003] -> Bus Creator5/3
  [FDDMEAS_2003001] -> Bus Creator3/1
  [FDDMEAS_2003002] -> Bus Creator3/2
  [FDDMEAS_2003003] -> Bus Creator3/3
  [FDDMEAS_2004001] -> Bus Creator4/1
  [FDDMEAS_2004002] -> Bus Creator4/2
  [FDDMEAS_2004003] -> Bus Creator4/3
  [FDDMEAS_2006001] -> Bus Creator6/1
  [FDDMEAS_2006002] -> Bus Creator6/2
  [FDDMEAS_2006003] -> Bus Creator6/3

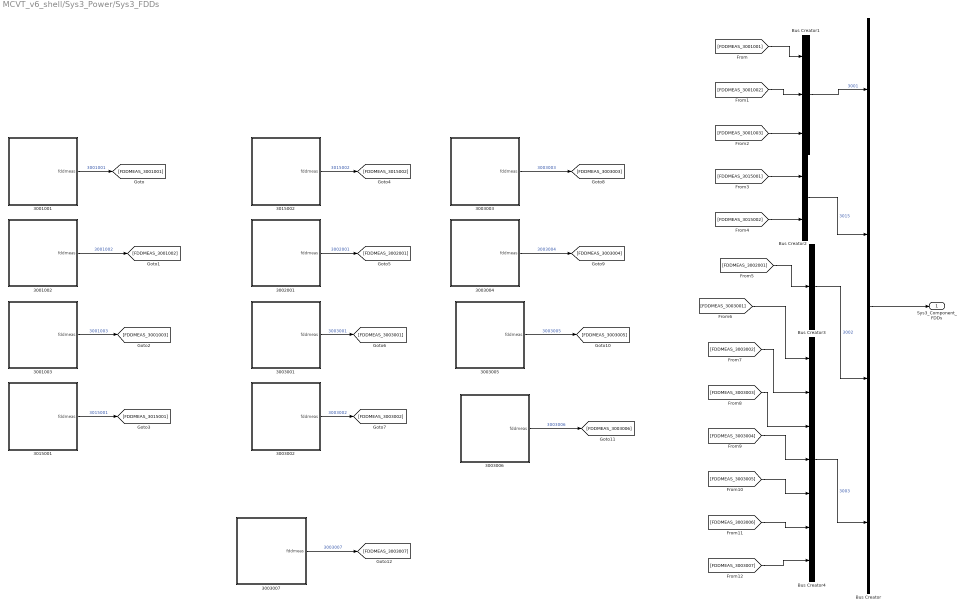
== system MCVT_v6_shell/Sys3_Power/Sys3_FDDs ==
  3001001 : MATLAB Function  TreatAsAtomicUnit=on
  3001002 : MATLAB Function  TreatAsAtomicUnit=on
  3001003 : MATLAB Function  TreatAsAtomicUnit=on
  3002001 : MATLAB Function  TreatAsAtomicUnit=on
  3003001 : MATLAB Function  TreatAsAtomicUnit=on
  3003002 : MATLAB Function  TreatAsAtomicUnit=on
  3003003 : MATLAB Function  TreatAsAtomicUnit=on
  3003004 : MATLAB Function  TreatAsAtomicUnit=on
  3003005 : MATLAB Function  TreatAsAtomicUnit=on
  3003006 : MATLAB Function  TreatAsAtomicUnit=on
  3003007 : MATLAB Function  TreatAsAtomicUnit=on
  3015001 : MATLAB Function  TreatAsAtomicUnit=on
  3015002 : MATLAB Function  TreatAsAtomicUnit=on
  Bus Creator : BusCreator  Inputs=4
  Bus Creator1 : BusCreator  Inputs=3
  Bus Creator2 : BusCreator  Inputs=2
  Bus Creator3 : BusCreator  Inputs=1
  Bus Creator4 : BusCreator  Inputs=7
  Sys3_Component_FDDs : Outport
  wires:
  3001002/1(fddmeas) -> [FDDMEAS_3001002]  "3001002"
  3002001/1(fddmeas) -> [FDDMEAS_3002001]  "3002001"
  3003002/1(fddmeas) -> [FDDMEAS_3003002]  "3003002"
  3015001/1(fddmeas) -> [FDDMEAS_3015001]  "3015001"
  3015002/1(fddmeas) -> [FDDMEAS_3015002]  "3015002"
  3003001/1(fddmeas) -> [FDDMEAS_3003001]  "3003001"
  3001003/1(fddmeas) -> [FDDMEAS_3001003]  "3001003"
  3003004/1(fddmeas) -> [FDDMEAS_3003004]  "3003004"
  3003003/1(fddmeas) -> [FDDMEAS_3003003]  "3003003"
  3001001/1(fddmeas) -> [FDDMEAS_3001001]  "3001001"
  Bus Creator/1 -> Sys3_Component_FDDs/1
  3003005/1(fddmeas) -> [FDDMEAS_3003005]  "3003005"
  3003006/1(fddmeas) -> [FDDMEAS_3003006]  "3003006"
  3003007/1(fddmeas) -> [FDDMEAS_3003007]  "3003007"
  [FDDMEAS_3001001] -> Bus Creator1/1
  [FDDMEAS_3001002] -> Bus Creator1/2
  [FDDMEAS_3001003] -> Bus Creator1/3
  [FDDMEAS_3015001] -> Bus Creator2/1
  [FDDMEAS_3015002] -> Bus Creator2/2
  Bus Creator1/1 -> Bus Creator/1  "3001"
  Bus Creator2/1 -> Bus Creator/2  "3015"
  Bus Creator4/1 -> Bus Creator/4  "3003"
  [FDDMEAS_3003001] -> Bus Creator4/1
  [FDDMEAS_3003002] -> Bus Creator4/2
  [FDDMEAS_3003003] -> Bus Creator4/3
  [FDDMEAS_3003004] -> Bus Creator4/4
  [FDDMEAS_3003005] -> Bus Creator4/5
  [FDDMEAS_3003006] -> Bus Creator4/6
  [FDDMEAS_3003007] -> Bus Creator4/7
  [FDDMEAS_3002001] -> Bus Creator3/1
  Bus Creator3/1 -> Bus Creator/3  "3002"

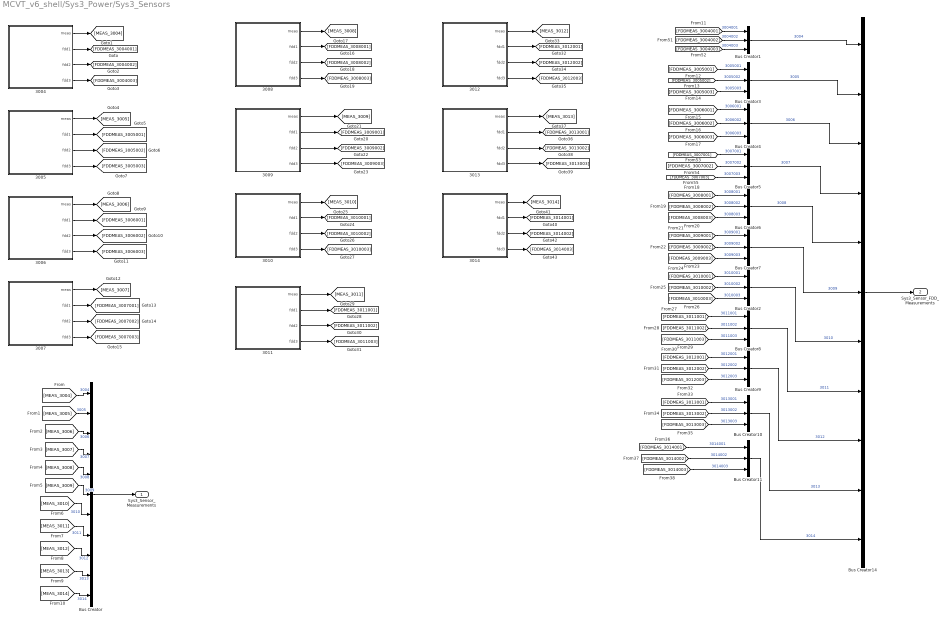
== system MCVT_v6_shell/Sys3_Power/Sys3_Sensors ==
  3004 : MATLAB Function  TreatAsAtomicUnit=on  SystemSampleTime=1/fz_3
  3005 : MATLAB Function  TreatAsAtomicUnit=on
  3006 : MATLAB Function  TreatAsAtomicUnit=on
  3007 : MATLAB Function  TreatAsAtomicUnit=on
  3008 : MATLAB Function  TreatAsAtomicUnit=on
  3009 : MATLAB Function  TreatAsAtomicUnit=on
  3010 : MATLAB Function  TreatAsAtomicUnit=on
  3011 : MATLAB Function  TreatAsAtomicUnit=on
  3012 : MATLAB Function  TreatAsAtomicUnit=on
  3013 : MATLAB Function  TreatAsAtomicUnit=on
  3014 : MATLAB Function  TreatAsAtomicUnit=on
  Bus Creator : BusCreator  Inputs=11
  Bus Creator{1..11} (11 alike) : BusCreator  Inputs=3
  Bus Creator14 : BusCreator  Inputs=11
  Sys3_Sensor_Measurements : Outport
  Sys3_Sensor_FDD_Measurements : Outport  Port=2
  wires:
  Bus Creator/1 -> Sys3_Sensor_Measurements/1
  3004/1(meas) -> [MEAS_3004]
  3004/2(fdd1) -> [FDDMEAS_3004001]
  3004/3(fdd2) -> [FDDMEAS_3004002]
  3004/4(fdd3) -> [FDDMEAS_3004003]
  3005/1(meas) -> [MEAS_3005]
  3005/2(fdd1) -> [FDDMEAS_3005001]
  3005/3(fdd2) -> [FDDMEAS_3005002]
  3005/4(fdd3) -> [FDDMEAS_3005003]
  3006/1(meas) -> [MEAS_3006]
  3006/2(fdd1) -> [FDDMEAS_3006001]
  3006/3(fdd2) -> [FDDMEAS_3006002]
  3006/4(fdd3) -> [FDDMEAS_3006003]
  3007/1(meas) -> [MEAS_3007]
  3007/2(fdd1) -> [FDDMEAS_3007001]
  3007/3(fdd2) -> [FDDMEAS_3007002]
  3007/4(fdd3) -> [FDDMEAS_3007003]
  3008/1(meas) -> [MEAS_3008]
  3008/2(fdd1) -> [FDDMEAS_3008001]
  3008/3(fdd2) -> [FDDMEAS_3008002]
  3008/4(fdd3) -> [FDDMEAS_3008003]
  3009/1(meas) -> [MEAS_3009]
  3009/2(fdd1) -> [FDDMEAS_3009001]
  3009/3(fdd2) -> [FDDMEAS_3009002]
  3009/4(fdd3) -> [FDDMEAS_3009003]
  3010/1(meas) -> [MEAS_3010]
  3010/2(fdd1) -> [FDDMEAS_3010001]
  3010/3(fdd2) -> [FDDMEAS_3010002]
  3010/4(fdd3) -> [FDDMEAS_3010003]
  3011/1(meas) -> [MEAS_3011]
  3011/2(fdd1) -> [FDDMEAS_3011001]
  3011/3(fdd2) -> [FDDMEAS_3011002]
  3011/4(fdd3) -> [FDDMEAS_3011003]
  3012/1(meas) -> [MEAS_3012]
  3012/2(fdd1) -> [FDDMEAS_3012001]
  3012/3(fdd2) -> [FDDMEAS_3012002]
  3012/4(fdd3) -> [FDDMEAS_3012003]
  3013/4(fdd3) -> [FDDMEAS_3013003]
  3013/3(fdd2) -> [FDDMEAS_3013002]
  3013/2(fdd1) -> [FDDMEAS_3013001]
  3013/1(meas) -> [MEAS_3013]
  3014/1(meas) -> [MEAS_3014]
  3014/2(fdd1) -> [FDDMEAS_3014001]
  3014/3(fdd2) -> [FDDMEAS_3014002]
  3014/4(fdd3) -> [FDDMEAS_3014003]
  [FDDMEAS_3004001] -> Bus Creator1/1  "3004001"
  [FDDMEAS_3004002] -> Bus Creator1/2  "3004002"
  [FDDMEAS_3004003] -> Bus Creator1/3  "3004003"
  [FDDMEAS_3005001] -> Bus Creator3/1  "3005001"
  [FDDMEAS_3005002] -> Bus Creator3/2  "3005002"
  [FDDMEAS_3005003] -> Bus Creator3/3  "3005003"
  [FDDMEAS_3006001] -> Bus Creator4/1  "3006001"
  [FDDMEAS_3006002] -> Bus Creator4/2  "3006002"
  [FDDMEAS_3006003] -> Bus Creator4/3  "3006003"
  [FDDMEAS_3007001] -> Bus Creator5/1  "3007001"
  [FDDMEAS_3007002] -> Bus Creator5/2  "3007002"
  [FDDMEAS_3007003] -> Bus Creator5/3  "3007003"
  Bus Creator1/1 -> Bus Creator14/1  "3004"
  Bus Creator3/1 -> Bus Creator14/2  "3005"
  Bus Creator4/1 -> Bus Creator14/3  "3006"
  Bus Creator5/1 -> Bus Creator14/4  "3007"
  Bus Creator6/1 -> Bus Creator14/5  "3008"
  Bus Creator7/1 -> Bus Creator14/6  "3009"
  Bus Creator2/1 -> Bus Creator14/7  "3010"
  Bus Creator8/1 -> Bus Creator14/8  "3011"
  Bus Creator9/1 -> Bus Creator14/9  "3012"
  Bus Creator10/1 -> Bus Creator14/10  "3013"
  Bus Creator11/1 -> Bus Creator14/11  "3014"
  Bus Creator14/1 -> Sys3_Sensor_FDD_Measurements/1
  [MEAS_3004] -> Bus Creator/1  "3004"
  [MEAS_3005] -> Bus Creator/2  "3005"
  [MEAS_3006] -> Bus Creator/3  "3006"
  [MEAS_3007] -> Bus Creator/4  "3007"
  [MEAS_3008] -> Bus Creator/5  "3008"
  [MEAS_3009] -> Bus Creator/6  "3009"
  [MEAS_3014] -> Bus Creator/11  "3014"
  [MEAS_3013] -> Bus Creator/10  "3013"
  [MEAS_3012] -> Bus Creator/9  "3012"
  [MEAS_3011] -> Bus Creator/8  "3011"
  [MEAS_3010] -> Bus Creator/7  "3010"
  [FDDMEAS_3008003] -> Bus Creator6/3  "3008003"
  [FDDMEAS_3008002] -> Bus Creator6/2  "3008002"
  [FDDMEAS_3008001] -> Bus Creator6/1  "3008001"
  [FDDMEAS_3009001] -> Bus Creator7/1  "3009001"
  [FDDMEAS_3009002] -> Bus Creator7/2  "3009002"
  [FDDMEAS_3009003] -> Bus Creator7/3  "3009003"
  [FDDMEAS_3010001] -> Bus Creator2/1  "3010001"
  [FDDMEAS_3010002] -> Bus Creator2/2  "3010002"
  [FDDMEAS_3010003] -> Bus Creator2/3  "3010003"
  [FDDMEAS_3011001] -> Bus Creator8/1  "3011001"
  [FDDMEAS_3011002] -> Bus Creator8/2  "3011002"
  [FDDMEAS_3011003] -> Bus Creator8/3  "3011003"
  [FDDMEAS_3012001] -> Bus Creator9/1  "3012001"
  [FDDMEAS_3012002] -> Bus Creator9/2  "3012002"
  [FDDMEAS_3012003] -> Bus Creator9/3  "3012003"
  [FDDMEAS_3013001] -> Bus Creator10/1  "3013001"
  [FDDMEAS_3013002] -> Bus Creator10/2  "3013002"
  [FDDMEAS_3013003] -> Bus Creator10/3  "3013003"
  [FDDMEAS_3014001] -> Bus Creator11/1  "3014001"
  [FDDMEAS_3014002] -> Bus Creator11/2  "3014002"
  [FDDMEAS_3014003] -> Bus Creator11/3  "3014003"

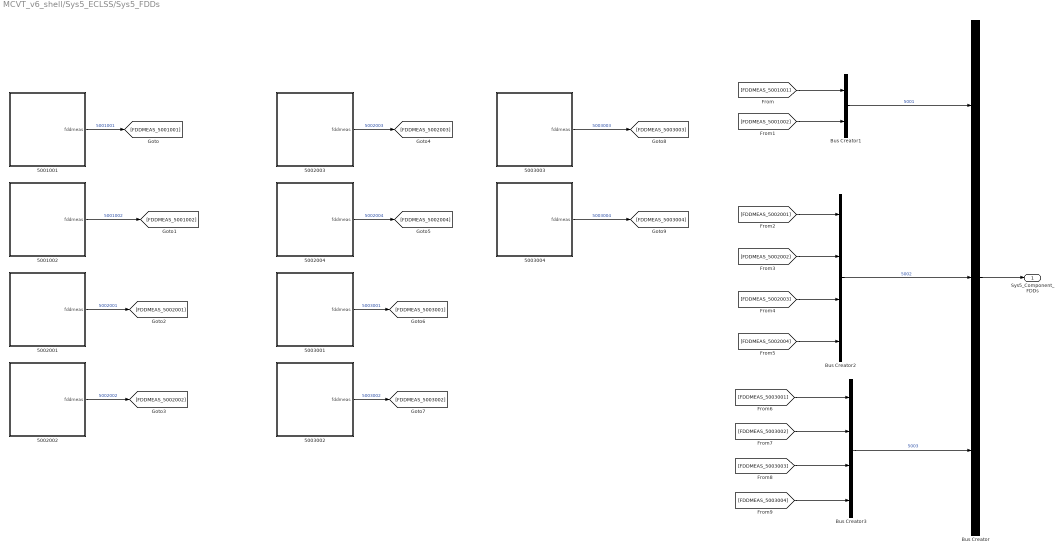
== system MCVT_v6_shell/Sys5_ECLSS/Sys5_FDDs ==
  5001001 : MATLAB Function  TreatAsAtomicUnit=on
  5001002 : MATLAB Function  TreatAsAtomicUnit=on
  5002001 : MATLAB Function  TreatAsAtomicUnit=on
  5002002 : MATLAB Function  TreatAsAtomicUnit=on
  5002003 : MATLAB Function  TreatAsAtomicUnit=on
  5002004 : MATLAB Function  TreatAsAtomicUnit=on
  5003001 : MATLAB Function  TreatAsAtomicUnit=on
  5003002 : MATLAB Function  TreatAsAtomicUnit=on
  5003003 : MATLAB Function  TreatAsAtomicUnit=on
  5003004 : MATLAB Function  TreatAsAtomicUnit=on
  Bus Creator : BusCreator  Inputs=3
  Bus Creator1 : BusCreator  Inputs=2
  Bus Creator2 : BusCreator  Inputs=4
  Bus Creator3 : BusCreator  Inputs=4
  Sys5_Component_FDDs : Outport
  wires:
  5001002/1(fddmeas) -> [FDDMEAS_5001002]  "5001002"
  5002004/1(fddmeas) -> [FDDMEAS_5002004]  "5002004"
  5003002/1(fddmeas) -> [FDDMEAS_5003002]  "5003002"
  5002002/1(fddmeas) -> [FDDMEAS_5002002]  "5002002"
  5002003/1(fddmeas) -> [FDDMEAS_5002003]  "5002003"
  5003001/1(fddmeas) -> [FDDMEAS_5003001]  "5003001"
  5002001/1(fddmeas) -> [FDDMEAS_5002001]  "5002001"
  5003004/1(fddmeas) -> [FDDMEAS_5003004]  "5003004"
  5003003/1(fddmeas) -> [FDDMEAS_5003003]  "5003003"
  5001001/1(fddmeas) -> [FDDMEAS_5001001]  "5001001"
  Bus Creator/1 -> Sys5_Component_FDDs/1
  [FDDMEAS_5001001] -> Bus Creator1/1
  [FDDMEAS_5001002] -> Bus Creator1/2
  Bus Creator1/1 -> Bus Creator/1  "5001"
  [FDDMEAS_5002001] -> Bus Creator2/1
  [FDDMEAS_5002002] -> Bus Creator2/2
  [FDDMEAS_5002003] -> Bus Creator2/3
  [FDDMEAS_5002004] -> Bus Creator2/4
  Bus Creator2/1 -> Bus Creator/2  "5002"
  [FDDMEAS_5003001] -> Bus Creator3/1
  [FDDMEAS_5003002] -> Bus Creator3/2
  [FDDMEAS_5003003] -> Bus Creator3/3
  [FDDMEAS_5003004] -> Bus Creator3/4
  Bus Creator3/1 -> Bus Creator/3  "5003"

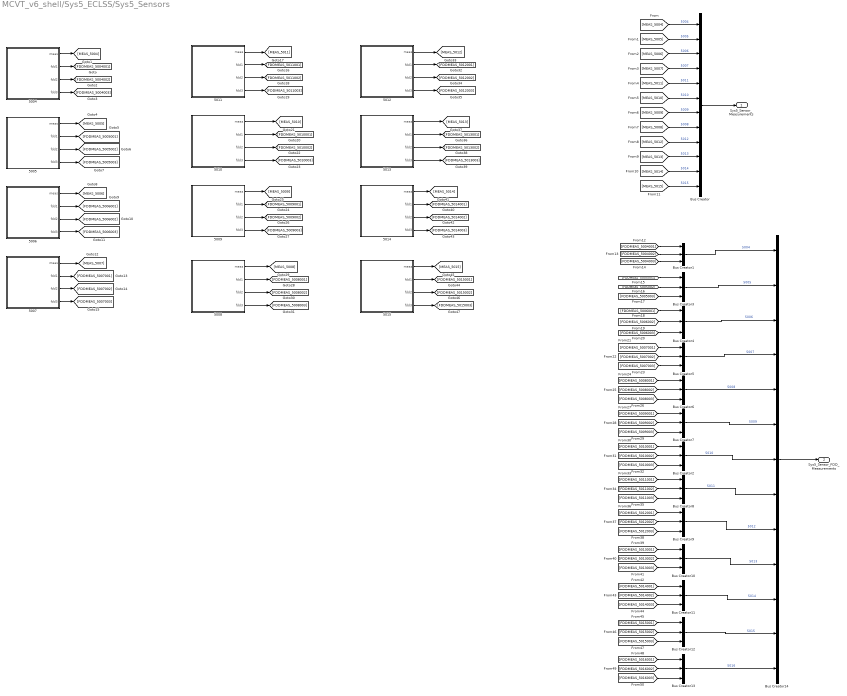
== system MCVT_v6_shell/Sys5_ECLSS/Sys5_Sensors ==
  5004 : MATLAB Function  TreatAsAtomicUnit=on
  5005 : MATLAB Function  TreatAsAtomicUnit=on
  5006 : MATLAB Function  TreatAsAtomicUnit=on
  5007 : MATLAB Function  TreatAsAtomicUnit=on
  5008 : MATLAB Function  TreatAsAtomicUnit=on
  5009 : MATLAB Function  TreatAsAtomicUnit=on
  5010 : MATLAB Function  TreatAsAtomicUnit=on
  5011 : MATLAB Function  TreatAsAtomicUnit=on
  5012 : MATLAB Function  TreatAsAtomicUnit=on
  5013 : MATLAB Function  TreatAsAtomicUnit=on
  5014 : MATLAB Function  TreatAsAtomicUnit=on
  5015 : MATLAB Function  TreatAsAtomicUnit=on
  Bus Creator : BusCreator  Inputs=12
  Bus Creator{1..13} (13 alike) : BusCreator  Inputs=3
  Bus Creator14 : BusCreator  Inputs=13
  Sys5_Sensor_Measurements : Outport
  Sys5_Sensor_FDD_Measurements : Outport  Port=2
  wires:
  Bus Creator/1 -> Sys5_Sensor_Measurements/1
  5004/1(meas) -> [MEAS_5004]
  5004/2(fdd1) -> [FDDMEAS_5004001]
  5004/3(fdd2) -> [FDDMEAS_5004002]
  5004/4(fdd3) -> [FDDMEAS_5004003]
  5005/1(meas) -> [MEAS_5005]
  5005/2(fdd1) -> [FDDMEAS_5005001]
  5005/3(fdd2) -> [FDDMEAS_5005002]
  5005/4(fdd3) -> [FDDMEAS_5005003]
  5006/1(meas) -> [MEAS_5006]
  5006/2(fdd1) -> [FDDMEAS_5006001]
  5006/3(fdd2) -> [FDDMEAS_5006002]
  5006/4(fdd3) -> [FDDMEAS_5006003]
  5007/1(meas) -> [MEAS_5007]
  5007/2(fdd1) -> [FDDMEAS_5007001]
  5007/3(fdd2) -> [FDDMEAS_5007002]
  5007/4(fdd3) -> [FDDMEAS_5007003]
  5011/1(meas) -> [MEAS_5011]
  5011/2(fdd1) -> [FDDMEAS_5011001]
  5011/3(fdd2) -> [FDDMEAS_5011002]
  5011/4(fdd3) -> [FDDMEAS_5011003]
  5010/1(meas) -> [MEAS_5010]
  5010/2(fdd1) -> [FDDMEAS_5010001]
  5010/3(fdd2) -> [FDDMEAS_5010002]
  5010/4(fdd3) -> [FDDMEAS_5010003]
  5009/1(meas) -> [MEAS_5009]
  5009/2(fdd1) -> [FDDMEAS_5009001]
  5009/3(fdd2) -> [FDDMEAS_5009002]
  5009/4(fdd3) -> [FDDMEAS_5009003]
  5008/1(meas) -> [MEAS_5008]
  5008/2(fdd1) -> [FDDMEAS_5008001]
  5008/3(fdd2) -> [FDDMEAS_5008002]
  5008/4(fdd3) -> [FDDMEAS_5008003]
  5012/1(meas) -> [MEAS_5012]
  5012/2(fdd1) -> [FDDMEAS_5012001]
  5012/3(fdd2) -> [FDDMEAS_5012002]
  5012/4(fdd3) -> [FDDMEAS_5012003]
  5013/4(fdd3) -> [FDDMEAS_5013003]
  5013/3(fdd2) -> [FDDMEAS_5013002]
  5013/2(fdd1) -> [FDDMEAS_5013001]
  5013/1(meas) -> [MEAS_5013]
  5014/1(meas) -> [MEAS_5014]
  5014/2(fdd1) -> [FDDMEAS_5014001]
  5014/3(fdd2) -> [FDDMEAS_5014002]
  5014/4(fdd3) -> [FDDMEAS_5014003]
  5015/1(meas) -> [MEAS_5015]
  5015/2(fdd1) -> [FDDMEAS_5015001]
  5015/3(fdd2) -> [FDDMEAS_5015002]
  5015/4(fdd3) -> [FDDMEAS_5015003]
  [MEAS_5004] -> Bus Creator/1  "5004"
  [MEAS_5005] -> Bus Creator/2  "5005"
  [MEAS_5006] -> Bus Creator/3  "5006"
  [MEAS_5007] -> Bus Creator/4  "5007"
  [MEAS_5011] -> Bus Creator/5  "5011"
  [MEAS_5010] -> Bus Creator/6  "5010"
  [MEAS_5009] -> Bus Creator/7  "5009"
  [MEAS_5008] -> Bus Creator/8  "5008"
  [MEAS_5012] -> Bus Creator/9  "5012"
  [MEAS_5013] -> Bus Creator/10  "5013"
  [MEAS_5014] -> Bus Creator/11  "5014"
  [MEAS_5015] -> Bus Creator/12  "5015"
  [FDDMEAS_5004001] -> Bus Creator1/1
  [FDDMEAS_5004002] -> Bus Creator1/2
  [FDDMEAS_5004003] -> Bus Creator1/3
  [FDDMEAS_5005001] -> Bus Creator3/1
  [FDDMEAS_5005002] -> Bus Creator3/2
  [FDDMEAS_5005003] -> Bus Creator3/3
  [FDDMEAS_5006001] -> Bus Creator4/1
  [FDDMEAS_5006002] -> Bus Creator4/2
  [FDDMEAS_5006003] -> Bus Creator4/3
  [FDDMEAS_5007001] -> Bus Creator5/1
  [FDDMEAS_5007002] -> Bus Creator5/2
  [FDDMEAS_5007003] -> Bus Creator5/3
  [FDDMEAS_5008001] -> Bus Creator6/1
  [FDDMEAS_5008002] -> Bus Creator6/2
  [FDDMEAS_5008003] -> Bus Creator6/3
  [FDDMEAS_5009001] -> Bus Creator7/1
  [FDDMEAS_5009002] -> Bus Creator7/2
  [FDDMEAS_5009003] -> Bus Creator7/3
  [FDDMEAS_5010003] -> Bus Creator2/3
  [FDDMEAS_5010002] -> Bus Creator2/2
  [FDDMEAS_5010001] -> Bus Creator2/1
  [FDDMEAS_5011003] -> Bus Creator8/3
  [FDDMEAS_5011002] -> Bus Creator8/2
  [FDDMEAS_5011001] -> Bus Creator8/1
  [FDDMEAS_5012003] -> Bus Creator9/3
  [FDDMEAS_5012002] -> Bus Creator9/2
  [FDDMEAS_5012001] -> Bus Creator9/1
  [FDDMEAS_5013003] -> Bus Creator10/3
  [FDDMEAS_5013002] -> Bus Creator10/2
  [FDDMEAS_5013001] -> Bus Creator10/1
  [FDDMEAS_5014003] -> Bus Creator11/3
  [FDDMEAS_5014002] -> Bus Creator11/2
  [FDDMEAS_5014001] -> Bus Creator11/1
  [FDDMEAS_5015003] -> Bus Creator12/3
  [FDDMEAS_5015002] -> Bus Creator12/2
  [FDDMEAS_5015001] -> Bus Creator12/1
  [FDDMEAS_5016003] -> Bus Creator13/3
  [FDDMEAS_5016002] -> Bus Creator13/2
  [FDDMEAS_5016001] -> Bus Creator13/1
  Bus Creator1/1 -> Bus Creator14/1  "5004"
  Bus Creator3/1 -> Bus Creator14/2  "5005"
  Bus Creator4/1 -> Bus Creator14/3  "5006"
  Bus Creator5/1 -> Bus Creator14/4  "5007"
  Bus Creator6/1 -> Bus Creator14/5  "5008"
  Bus Creator7/1 -> Bus Creator14/6  "5009"
  Bus Creator2/1 -> Bus Creator14/7  "5010"
  Bus Creator8/1 -> Bus Creator14/8  "5011"
  Bus Creator9/1 -> Bus Creator14/9  "5012"
  Bus Creator10/1 -> Bus Creator14/10  "5013"
  Bus Creator11/1 -> Bus Creator14/11  "5014"
  Bus Creator12/1 -> Bus Creator14/12  "5015"
  Bus Creator13/1 -> Bus Creator14/13  "5016"
  Bus Creator14/1 -> Sys5_Sensor_FDD_Measurements/1

== system MCVT_v6_shell/Sys8_Interior_Environment/Sys8_FDDs ==
  8001001 : MATLAB Function  TreatAsAtomicUnit=on
  Bus Creator : BusCreator  Inputs=1
  Sys8_Component_FDD_Suite : Outport
  wires:
  8001001/1(fddmeas) -> [FDDMEAS_8001001]  "8001001"
  [FDDMEAS_8001001] -> Bus Creator/1
  Bus Creator/1 -> Sys8_Component_FDD_Suite/1  "8001"

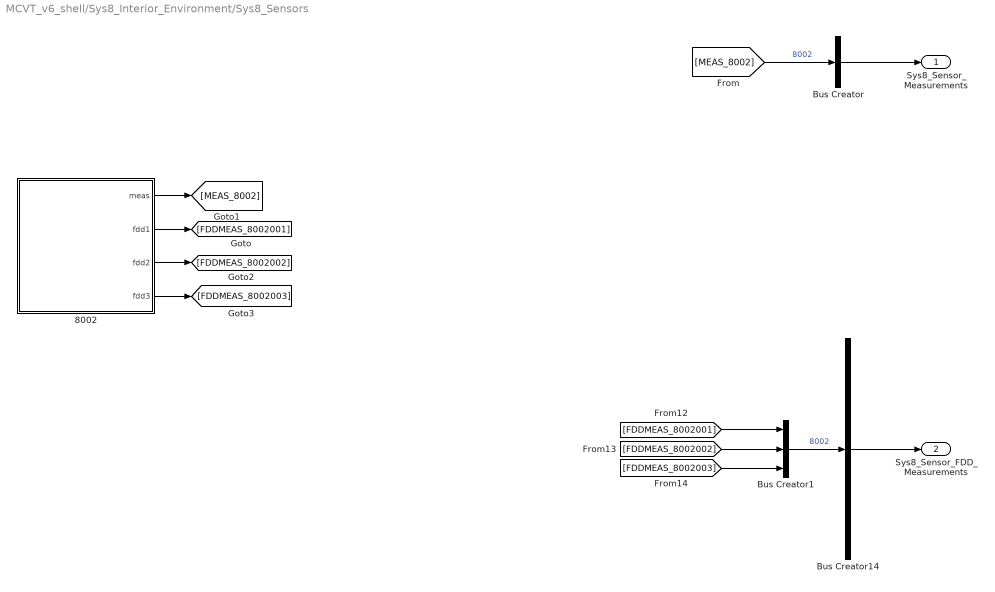
== system MCVT_v6_shell/Sys8_Interior_Environment/Sys8_Sensors ==
  8002 : MATLAB Function  TreatAsAtomicUnit=on
  Bus Creator : BusCreator  Inputs=1
  Bus Creator1 : BusCreator  Inputs=3
  Bus Creator14 : BusCreator  Inputs=1
  Sys8_Sensor_Measurements : Outport
  Sys8_Sensor_FDD_Measurements : Outport  Port=2
  wires:
  Bus Creator/1 -> Sys8_Sensor_Measurements/1
  8002/1(meas) -> [MEAS_8002]
  8002/2(fdd1) -> [FDDMEAS_8002001]
  8002/3(fdd2) -> [FDDMEAS_8002002]
  8002/4(fdd3) -> [FDDMEAS_8002003]
  [MEAS_8002] -> Bus Creator/1  "8002"
  [FDDMEAS_8002001] -> Bus Creator1/1
  [FDDMEAS_8002002] -> Bus Creator1/2
  [FDDMEAS_8002003] -> Bus Creator1/3
  Bus Creator1/1 -> Bus Creator14/1  "8002"
  Bus Creator14/1 -> Sys8_Sensor_FDD_Measurements/1

== matlab function MCVT_v6_shell/Sys5_ECLSS/Sys5_FDDs/5001001 ==
  settings: updateMethod=DISCRETE  sampleTime=1/fz_5
  data: fddmeas output
function fddmeas = FDD_model()

    fddmeas = rand(1,1);
    
end

== matlab function MCVT_v6_shell/Sys5_ECLSS/Sys5_Sensors/5009 ==
  settings: updateMethod=DISCRETE  sampleTime=1/fz_5
  data: meas output; fdd1 output; fdd2 output; fdd3 output
function [meas, fdd1, fdd2, fdd3] = Sensor_Model()
    
    meas = rand();
    fdd1 = randi([0 1]);
    fdd2 = rand();
    fdd3 = randi([0 1]);
    
end

== matlab function MCVT_v6_shell/Sys5_ECLSS/Sys5_Sensors/5010 ==
  settings: updateMethod=DISCRETE  sampleTime=1/fz_5
  data: meas output; fdd1 output; fdd2 output; fdd3 output
function [meas, fdd1, fdd2, fdd3] = Sensor_Model()
    
    meas = rand();
    fdd1 = randi([0 1]);
    fdd2 = rand();
    fdd3 = randi([0 1]);
    
end

== matlab function MCVT_v6_shell/Sys5_ECLSS/Sys5_Sensors/5011 ==
  settings: updateMethod=DISCRETE  sampleTime=1/fz_5
  data: meas output; fdd1 output; fdd2 output; fdd3 output
function [meas, fdd1, fdd2, fdd3] = Sensor_Model()
    
    meas = rand();
    fdd1 = randi([0 1]);
    fdd2 = rand();
    fdd3 = randi([0 1]);
    
end

== matlab function MCVT_v6_shell/Sys5_ECLSS/Sys5_Sensors/5012 ==
  settings: updateMethod=DISCRETE  sampleTime=1/fz_5
  data: meas output; fdd1 output; fdd2 output; fdd3 output
function [meas, fdd1, fdd2, fdd3] = Sensor_Model()
    
    meas = rand();
    fdd1 = randi([0 1]);
    fdd2 = rand();
    fdd3 = randi([0 1]);
    
end

== matlab function MCVT_v6_shell/Sys5_ECLSS/Sys5_Sensors/5013 ==
  settings: updateMethod=DISCRETE  sampleTime=1/fz_5
  data: meas output; fdd1 output; fdd2 output; fdd3 output
function [meas, fdd1, fdd2, fdd3] = Sensor_Model()
    
    meas = rand();
    fdd1 = randi([0 1]);
    fdd2 = rand();
    fdd3 = randi([0 1]);
    
end

== matlab function MCVT_v6_shell/Sys5_ECLSS/Sys5_Sensors/5014 ==
  settings: updateMethod=DISCRETE  sampleTime=1/fz_5
  data: meas output; fdd1 output; fdd2 output; fdd3 output
function [meas, fdd1, fdd2, fdd3] = Sensor_Model()
    
    meas = rand();
    fdd1 = randi([0 1]);
    fdd2 = rand();
    fdd3 = randi([0 1]);
    
end

== matlab function MCVT_v6_shell/Sys5_ECLSS/Sys5_FDDs/5001002 ==
  settings: updateMethod=DISCRETE  sampleTime=1/fz_5
  data: fddmeas output
function fddmeas = FDD_model()

    fddmeas = rand(1,1);
    
end

== matlab function MCVT_v6_shell/Sys5_ECLSS/Sys5_Sensors/5004 ==
  settings: updateMethod=DISCRETE  sampleTime=1/fz_5
  data: meas output; fdd1 output; fdd2 output; fdd3 output
function [meas, fdd1, fdd2, fdd3] = Sensor_Model()
    
    meas = rand();
    fdd1 = randi([0 1]);
    fdd2 = rand();
    fdd3 = randi([0 1]);
    
end

== matlab function MCVT_v6_shell/Sys5_ECLSS/Sys5_Sensors/5015 ==
  settings: updateMethod=DISCRETE  sampleTime=1/fz_5
  data: meas output; fdd1 output; fdd2 output; fdd3 output
function [meas, fdd1, fdd2, fdd3] = Sensor_Model()
    
    meas = rand();
    fdd1 = randi([0 1]);
    fdd2 = rand();
    fdd3 = randi([0 1]);
    
end

== matlab function MCVT_v6_shell/Sys11_SPL/Sys11_FDDs/11001001 ==
  settings: updateMethod=DISCRETE  sampleTime=1/fz_11
  data: fddmeas output
function fddmeas = FDD_model()

    fddmeas = rand(1,1);
    
end

== matlab function MCVT_v6_shell/Sys2_Structure/Sys2_FDDs/2001001 ==
  settings: updateMethod=DISCRETE  sampleTime=1/fz_2
  data: fddmeas output
function fddmeas = FDD_model()

    fddmeas = rand(1,1);
    
end

== matlab function MCVT_v6_shell/Sys3_Power/Sys3_FDDs/3001001 ==
  settings: updateMethod=DISCRETE  sampleTime=1/fz_3
  data: fddmeas output
function fddmeas = FDD_model()

    fddmeas = rand(4,1);
    
end

== matlab function MCVT_v6_shell/Sys3_Power/Sys3_FDDs/3001002 ==
  settings: updateMethod=DISCRETE  sampleTime=1/fz_3
  data: fddmeas output
function fddmeas = FDD_model()

    fddmeas = rand(1,1);
    
end

== matlab function MCVT_v6_shell/Sys3_Power/Sys3_FDDs/3001003 ==
  settings: updateMethod=DISCRETE  sampleTime=1/fz_3
  data: fddmeas output
function fddmeas = FDD_model()

    fddmeas = rand(1,1);
    
end

== matlab function MCVT_v6_shell/Sys3_Power/Sys3_FDDs/3015001 ==
  settings: updateMethod=DISCRETE  sampleTime=1/fz_3
  data: fddmeas output
function fddmeas = FDD_model()

    fddmeas = rand(1,1);
    
end

== matlab function MCVT_v6_shell/Sys3_Power/Sys3_FDDs/3015002 ==
  settings: updateMethod=DISCRETE  sampleTime=1/fz_3
  data: fddmeas output
function fddmeas = FDD_model()

    fddmeas = rand(1,1);
    
end

== matlab function MCVT_v6_shell/Sys5_ECLSS/Sys5_FDDs/5002001 ==
  settings: updateMethod=DISCRETE  sampleTime=1/fz_5
  data: fddmeas output
function fddmeas = FDD_model()

    fddmeas = rand(1,1);
    
end

== matlab function MCVT_v6_shell/Sys3_Power/Sys3_FDDs/3002001 ==
  settings: updateMethod=DISCRETE  sampleTime=1/fz_3
  data: fddmeas output
function fddmeas = FDD_model()

    fddmeas = rand(1,1);
    
end

== matlab function MCVT_v6_shell/Sys8_Interior_Environment/Sys8_FDDs/8001001 ==
  settings: updateMethod=DISCRETE  sampleTime=1/fz_8
  data: fddmeas output
function fddmeas = FDD_model()

    fddmeas = rand(1,1);
    
end

== matlab function MCVT_v6_shell/Sys3_Power/Sys3_FDDs/3003001 ==
  settings: updateMethod=DISCRETE  sampleTime=1/fz_3
  data: fddmeas output
function fddmeas = FDD_model()

    fddmeas = rand(1,1);
    
end

== matlab function MCVT_v6_shell/Sys8_Interior_Environment/Sys8_Sensors/8002 ==
  settings: updateMethod=DISCRETE  sampleTime=1/fz_8
  data: meas output; fdd1 output; fdd2 output; fdd3 output
function [meas, fdd1, fdd2, fdd3] = Sensor_Model()
    
    meas = rand();
    fdd1 = randi([0 1]);
    fdd2 = rand();
    fdd3 = randi([0 1]);
    
end

== matlab function MCVT_v6_shell/Sys3_Power/Sys3_FDDs/3003002 ==
  settings: updateMethod=DISCRETE  sampleTime=1/fz_3
  data: fddmeas output
function fddmeas = FDD_model()

    fddmeas = rand(1,1);
    
end
